simulink model "SCCBoostConverter_v2"  (R2018a)
settings: Solver=VariableStepAuto  StartTime=0.0  StopTime=0.5  RelTol=1e-3  AbsTol=1e-3  EnableMultiTasking=on
undefined symbols (not defined in the file or in its folder): D
libraries: powerlib x15, powerlib_meascontrol x2
settings Model: Creator=snow_  LastModifiedBy=snow_
settings SolverCC: AutoScaleAbsTol=off
settings DataIOCC: LimitDataPoints=on  MaxDataPoints=10000
settings OptimizationCC: LifeSpan=inf
settings DebuggingCC: AllowSymbolicDim=off  SFUnexpectedBacktrackingDiag=warning  SFNoUnconditionalDefaultTransitionDiag=warning  SFExecutionAtInitializationDiag=none
settings CodeAppCC: StateflowObjectComments=on
settings GRTTargetCC: TargetLangStandard=C89/C90 (ANSI)  GeneratePreprocessorConditionals=Disable all
settings ConfigComp: CovMetricSettings=dw  CovHtmlReporting=on  CovSaveCumulativeToWorkspaceVar=on  CovSaveSingleToWorkspaceVar=on  CovExternalEMLEnable=off  CovSFcnEnable=off
settings SimscapeCC: SimscapeLogType=all  SimscapeLogDataHistory=10000

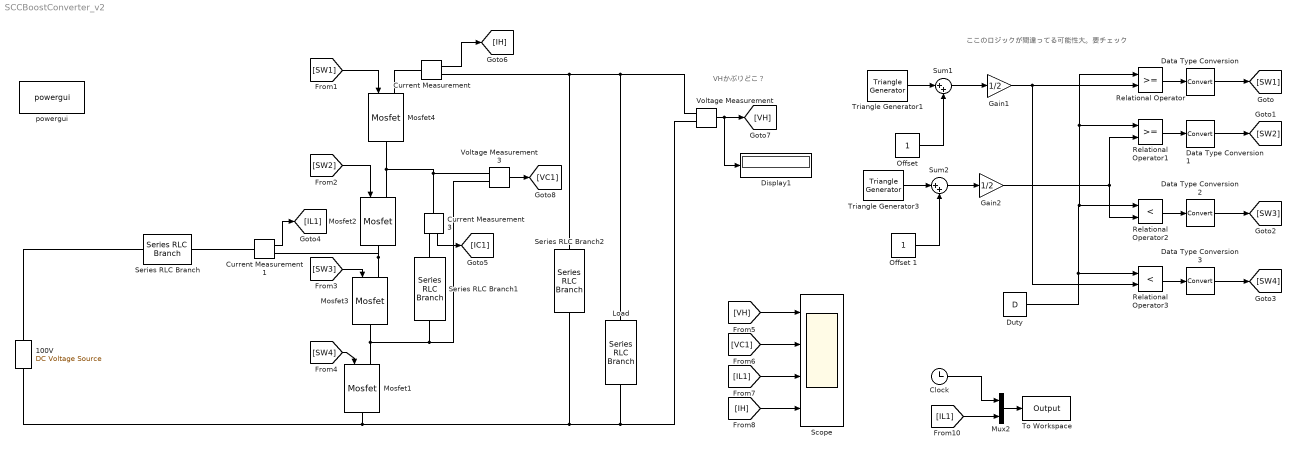
== system SCCBoostConverter_v2 ==
  note: ここのロジックが間違ってる可能性大。要チェック
  note: VHかぶりどこ？
  100V : powerlib/Electrical Sources/DC Voltage Source  Amplitude=100  Measurements=None
  Clock : Clock
  Current Measurement : powerlib/Measurements/Current Measurement  PhasorSimulation=off  OutputType=Complex  PSBequivalent=0
  Current Measurement1 : powerlib/Measurements/Current Measurement  PhasorSimulation=off  OutputType=Complex  PSBequivalent=0
  Current Measurement3 : powerlib/Measurements/Current Measurement  PhasorSimulation=off  OutputType=Complex  PSBequivalent=0
  Data Type Conversion{,1..3} (4 alike) : DataTypeConversion
  Display1 : Display
  "Duty " : Constant  Value=D
  Gain1 : Gain  Gain=1/2
  Gain2 : Gain  Gain=1/2
  Load : powerlib/Elements/Series RLC Branch  LConnTagsString=__new0  RConnTagsString=__new0  BranchType=R  Resistance=1/(1-D)*200/100  Inductance=20e-6  SetiL0=off  InitialCurrent=0  Capacitance=1e-6  Setx0=off  InitialVoltage=0  Measurements=None
      settings: AttributesFormatString=R = %<Resistance> Ohm
  Mosfet{1..4} (4 alike) : powerlib/Power Electronics/Mosfet  Ron=0.005  Lon=0  Rd=0.005  Vfd=0  IC=0  Rs=1e5  Cs=inf  Measurements=off
  Mux2 : Mux  Inputs=2
  "Offset " : Constant
  Offset 1 : Constant
  Relational Operator : RelationalOperator  OutDataTypeStr=boolean  RndMeth=Simplest
  Relational Operator1 : RelationalOperator  OutDataTypeStr=boolean  RndMeth=Simplest
  Relational Operator2 : RelationalOperator  Operator=<  OutDataTypeStr=boolean  RndMeth=Simplest
  Relational Operator3 : RelationalOperator  Operator=<  OutDataTypeStr=boolean  RndMeth=Simplest
  Scope : Scope  NumInputPorts=4
  Series RLC Branch : powerlib/Elements/Series RLC Branch  LConnTagsString=__new0  RConnTagsString=__new0  BranchType=L  Resistance=24e-3  Inductance=10e-6  SetiL0=off  InitialCurrent=0  Capacitance=1e-6  Setx0=off  InitialVoltage=0  Measurements=None
      settings: AttributesFormatString=|
      | L=%<Inductance> H
      | R=%<Resistance> Ohm
  Series RLC Branch1 : powerlib/Elements/Series RLC Branch  LConnTagsString=__new0  RConnTagsString=__new0  BranchType=C  Resistance=24e-3  Inductance=1000e-6  SetiL0=off  InitialCurrent=0  Capacitance=30e-6  Setx0=off  InitialVoltage=0  Measurements=None
      settings: AttributesFormatString=C=%<Capacitance>
  Series RLC Branch2 : powerlib/Elements/Series RLC Branch  LConnTagsString=__new0  RConnTagsString=__new0  BranchType=C  Resistance=24e-3  Inductance=1000e-6  SetiL0=off  InitialCurrent=0  Capacitance=1000e-6  Setx0=off  InitialVoltage=0  Measurements=None
      settings: AttributesFormatString=C=%<Capacitance>
  Sum1 : Sum  Inputs=|++
  Sum2 : Sum  Inputs=|++
  To Workspace : ToWorkspace  VariableName=Output  SampleTime=1e-6
  Triangle Generator1 : powerlib_meascontrol/Pulse & Signal Generators/Triangle Generator  Freq=20e3  Phase=0  Ts=0
      settings: AttributesFormatString=Freq = %<Freq> Hz
  Triangle Generator3 : powerlib_meascontrol/Pulse & Signal Generators/Triangle Generator  Freq=20e3  Phase=180  Ts=0
      settings: AttributesFormatString=Freq = %<Freq> Hz
  Voltage Measurement : powerlib/Measurements/Voltage Measurement  PhasorSimulation=off  OutputType=Complex  PSBequivalent=0
  Voltage Measurement3 : powerlib/Measurements/Voltage Measurement  PhasorSimulation=off  OutputType=Complex  PSBequivalent=0
  powergui : powerlib/powergui  Priority=1  SimulationMode=Continuous  SampleTime=50e-6  frequency=60  Iterations=50  frequencyindice=0  Pbase=100e6  ErrMax=1e-4  UnitsV=kV  UnitsW=MW  buscounter=0  FunctionMessages=off  echomessages=off  EnableUseOfTLC=off  CurrentSourceSwitches=off  DisableSnubberDevices=off  DisableRonSwitches=off  DisableVfSwitches=off  DisplayEquations=off  SolverType=Tustin/Backward Euler (TBE)  Interpol=off  ExternalGateDelay=off  methode=off  Ts=100  x0status=blocks  SPID=on  SwTol=0  HookPort=off  RestoreLinks=warning  ResistiveCurrentMeasurement=off  Frange=[0:2:500]  Ylog=off  Xlog=on  ShowGrid=off  save=off  variable=ZData  structure=0  ZoomFFT=off  StartTime=0.0  cycles=1  DisplayStyle=1  fundamental=60  FreqAxis=off  MaxFrequency=1000  frequencyindicesteady=1  RmsSteady=1  display=off
  wires:
  Clock/1 -> Mux2/1
  "Offset "/1 -> Sum1/2
  Sum1/1 -> Gain1/1
  Relational Operator/1 -> Data Type Conversion/1
  Relational Operator1/1 -> Data Type Conversion1/1
  Gain1/1 -> Relational Operator3/2, Relational Operator/2
  "Duty "/1 -> Relational Operator3/1, Relational Operator2/1, Relational Operator1/1, Relational Operator/1
  Triangle Generator1/1 -> Sum1/1
  [IL1] -> Mux2/2
  Data Type Conversion3/1 -> [SW4]
  Data Type Conversion/1 -> [SW1]
  Relational Operator3/1 -> Data Type Conversion3/1
  Data Type Conversion2/1 -> [SW3]
  Relational Operator2/1 -> Data Type Conversion2/1
  Mux2/1 -> To Workspace/1
  Data Type Conversion1/1 -> [SW2]
  Triangle Generator3/1 -> Sum2/1
  Offset 1/1 -> Sum2/2
  Sum2/1 -> Gain2/1
  Gain2/1 -> Relational Operator2/2, Relational Operator1/2
  [SW1] -> Mosfet4/1
  [SW2] -> Mosfet2/1
  [SW3] -> Mosfet3/1
  [SW4] -> Mosfet1/1
  Current Measurement1/1 -> [IL1]
  Current Measurement3/1 -> [IC1]
  Current Measurement/1 -> [IH]
  Voltage Measurement/1 -> [VH], Display1/1
  Voltage Measurement3/1 -> [VC1]
  [VH] -> Scope/1
  [IL1] -> Scope/3
  [IH] -> Scope/4
  [VC1] -> Scope/2
  connections:
  Series RLC Branch/LConn1 -- 100V/RConn1
  Mosfet1/LConn1 -- Series RLC Branch1/RConn1 -- Voltage Measurement3/LConn2 -- Mosfet3/RConn1
  Mosfet2/LConn1 -- Voltage Measurement3/LConn1 -- Current Measurement3/LConn1 -- Mosfet4/RConn1
  Current Measurement/RConn1 -- Voltage Measurement/LConn1 -- Load/LConn1 -- Series RLC Branch2/LConn1
  Voltage Measurement/LConn2 -- Load/RConn1 -- 100V/LConn1 -- Mosfet1/RConn1 -- Series RLC Branch2/RConn1
  Mosfet4/LConn1 -- Current Measurement/LConn1
  Series RLC Branch/RConn1 -- Current Measurement1/LConn1
  Mosfet2/RConn1 -- Mosfet3/LConn1 -- Current Measurement1/RConn1
  Current Measurement3/RConn1 -- Series RLC Branch1/LConn1
